simulink model "afe_abc_inv_psm_2mods"  (R2025b)
settings: Solver=ode1  StartTime=0.0  StopTime=simlength  FixedStep=tc  MaxStep=tc
values from neighbouring files (symbols this model uses):
  Adrso = eye(2) + Arso*ts_afe    [init_model.m]
  afe_pwm_phase_shift_mod1 = 0    [init_model.m]
  afe_pwm_phase_shift_mod2 = 0    [init_model.m]
  Aresd = eye(2) + Ares*ts_afe    [init_model.m]
  Bresd = Bres*ts_afe    [init_model.m]
  Cresd = Cres    [init_model.m]
  Crso = [1 0]    [init_model.m]
  CTRPIFF_CLIP_RELEASE = 0.001    [init_model.m]
  dead_time_AFE = 3e-6    (= 3e-06)    [init_model.m]
  dead_time_INV = 3e-6    (= 3e-06)    [init_model.m]
  deepNEGeta = 0.5    [init_model.m]
  deepNEGxi = 0    [init_model.m]
  deepPOSxi = 0.5    [init_model.m]
  emf_fb_p = 0.2    [init_model.m]
  emf_fb_p_ccaller_1 = emf_fb_p    (= 0.2)    [init_model.m]
  emf_fb_p_ccaller_2 = emf_fb_p    (= 0.2)    [init_model.m]
  emf_p = emf_fb_p*4/10    (= 0.08)    [init_model.m]
  emf_p_ccaller_1 = emf_fb_p_ccaller_1*4/10    (= 0.08)    [init_model.m]
  emf_p_ccaller_2 = emf_fb_p_ccaller_2*4/10    (= 0.08)    [init_model.m]
  fPWM_AFE = 4e3    (= 4000)    [init_model.m]
  fPWM_INV = fPWM_AFE    (= 4000)    [init_model.m]
  g0_161Hz = fcut_161Hz_flt * ts_afe * 2*pi    (= 0.126449104307)    [init_model.m]
  g0_1Hz = fcut_1Hz_flt * ts_afe * 2*pi    (= 0.000785398163397)    [init_model.m]
  g0_500Hz = fcut_500Hz_flt * ts_afe * 2*pi    (= 0.392699081699)    [init_model.m]
  g1_161Hz = 1 - g0_161Hz    (= 0.873550895693)    [init_model.m]
  g1_1Hz = 1 - g0_1Hz    (= 0.999214601837)    [init_model.m]
  g1_500Hz = 1 - g0_500Hz    (= 0.607300918301)    [init_model.m]
  i_grid_neg_eta_lim = 0.5    [init_model.m]
  i_grid_neg_eta_red_lim = 0.1    [init_model.m]
  i_grid_neg_xi_lim = 0.5    [init_model.m]
  i_grid_neg_xi_red_lim = 0.1    [init_model.m]
  i_grid_pos_eta_lim = 1    [init_model.m]
  i_grid_pos_eta_red_lim = 0.1    [init_model.m]
  id_lim = 0.35    [init_model.m]
  ieta_neg_ref_lim = 0.5    [init_model.m]
  ieta_pos_ref_lim = 1.0    (= 1)    [init_model.m]
  Igrid_phase_normalization_factor = 250e3/Vphase2/3/0.9*sqrt(2)    [init_model.m]
  inv_pwm_phase_shift_mod1 = 0    [init_model.m]
  iq_lim = 1.4    [init_model.m]
  ixi_pos_ref_lim = 1.6    [init_model.m]
  k_frt_ref = 2    [init_model.m]
  kg = Kobs(1)    [init_model.m]
  ki_afe = 45    [init_model.m]
  ki_align = 0.1    [init_model.m]
  ki_i = 18    [init_model.m]
  ki_rc_neg_grid = ki_rc_grid    (= 35)    [init_model.m]
  ki_rc_pos_grid = ki_rc_grid    (= 35)    [init_model.m]
  ki_vs = 35    [init_model.m]
  ki_w = 18    [init_model.m]
  kp_afe = 0.6    [init_model.m]
  kp_align = 0.6    [init_model.m]
  kp_i = 0.25    [init_model.m]
  kp_rc_neg_grid = kp_rc_grid    (= 0.35)    [init_model.m]
  kp_rc_pos_grid = kp_rc_grid    (= 0.35)    [init_model.m]
  kp_vs = 0.85    [init_model.m]
  kp_w = 2.5    [init_model.m]
  kw = Kobs(2)    [init_model.m]
  l1 = Kd(2)    [init_model.m]
  l2 = Kd(1)    [init_model.m]
  Ldrso = acker(Adrso',Crso',polesdrso)'    [init_model.m]
  lim_down_align = -0.2    [init_model.m]
  lim_up_align = 0.2    [init_model.m]
  mavarage_filter_frequency_base_order = 2    [init_model.m]
  motorc_m_scale = 2/3*Vdc_bez/ubez    [init_model.m]
  n1 = rms_perios/f_grid/ts_afe    [init_model.m]
  n10 = rms_perios/f_grid/ts_afe    [init_model.m]
  number_of_modules = 2    [init_model.m]
  omega_m_sim = omega_m_bez    [init_model.m]
  pll_i1 = 80    [init_model.m]
  pll_i1_ddsrt = pll_i1/2    (= 40)    [init_model.m]
  pll_p = 1    [init_model.m]
  pll_p_ddsrt = pll_p/2    (= 0.5)    [init_model.m]
  pll_p_frt = 0.2    [init_model.m]
  settle_time = 0.15    [init_model.m]
  simlength = 2    [init_model.m]
  start_time_LVRT = 2.0    (= 2)    [init_model.m]
  tc = ts_afe/200    (= 6.25e-07)    [init_model.m]
  time_aux_power_supply_fault = 1e3    (= 1000)    [init_model.m]
  time_gain_afe_module_1 = 1.0    (= 1)    [init_model.m]
  time_gain_afe_module_2 = 1.0    (= 1)    [init_model.m]
  time_gain_inv_module_1 = 1.0    (= 1)    [init_model.m]
  time_gain_inv_module_2 = 1.0    (= 1)    [init_model.m]
  time_phase_fault = 1e3    (= 1000)    [init_model.m]
  time_start_motor_control = 0.035    [init_model.m]
  transmission_delay = 125e-6*2    (= 0.00025)    [init_model.m]
  ts_afe = 1/fPWM_AFE/2    (= 0.000125)    [init_model.m]
  ts_inv = 1/fPWM_INV/2    (= 0.000125)    [init_model.m]
  Vdc_norm_ref = Vdc_ref/Vdc_nom    [init_model.m]
  Vdc_ref = 1070    [init_model.m]
  Vgrid_phase_normalization_factor = Vphase2*sqrt(2)    [init_model.m]
  w_grid = 2*pi*f_grid    [init_model.m]
undefined symbols (not defined in the file or in its folder): Amplitude_U, Amplitude_V, Amplitude_W, end_time_LVRT, ibez, La, Lb, Ld_norm, Lq_norm, Ls_norm, magnitude, omega_bez, omega_grid_emulator_nom, omega_grid_nom, omega_m_bez, Phase_shift, psi_bez, psi_m, psi_m_norm, rpm_base, rpm_bez, Rs, Rs_norm, t_ramp, tau_bez, torque_base, ubez, ugrid_factor, V_phase_normalization_factor, Vdc_bez, Vemu_ref_norm, vn_eta_pu, vn_xi_pu, vp_xi_pu
libraries: fl_lib x215, nesl_utility x107, simulink x22, cstblocks x20, threephase_inductor_lib x4, single_phase_transformer_lib x3, flexshaft_lib x1, psm x1
(part 12 of 19)

== system afe_abc_inv_psm_2mods/afe_abc_inv_psm_mod2/AFE_control/afe_control/grid_voltage_phase_lock_loops/DDSRF-PLL/pll_stageB ==
  u_grid_pos_xi : Inport
  u_grid_pos_eta : Inport  Port=2
  -2<x<2 : Saturate  UpperLimit=2  LowerLimit=-2
  Constant2 : Constant
  Constant3 : Constant  Value=0
  Constant4 : Constant  Value=omega_grid_nom
  Constant5 : Constant
  Constant6 : Constant  Value=-1
  Math Function : Math  Operator=magnitude^2  SignedPower=on
  Math Function2 : Math  Operator=magnitude^2  SignedPower=on
  Product{,1..3} (4 alike) : Product  RndMeth=Zero
  Sqrt : Sqrt
  Sum : Sum  Inputs=|-+
  Sum1 : Sum  Inputs=|-+
  Sum2 : Sum  Inputs=|++
  Sum3 : Sum  SaturateOnIntegerOverflow=on
  Sum4 : Sum  SaturateOnIntegerOverflow=on
  Sum5 : Sum  Inputs=++|
  Switch : Switch  Criteria=u2 > Threshold  SaturateOnIntegerOverflow=off  InputSameDT=off
  To Workspace5 : ToWorkspace  VariableName=vgrid_xi_pll_pos  SampleTime=-1
      settings: MaxDataPoints=Ns_afe
  To Workspace6 : ToWorkspace  VariableName=vgrid_eta_pll_pos  SampleTime=-1
      settings: MaxDataPoints=Ns_afe
  Unit Delay1 : UnitDelay  SampleTime=-1  HasFrameUpgradeWarning=on
  Unit Delay2 : UnitDelay  SampleTime=-1  HasFrameUpgradeWarning=on
  Unit Delay4 : UnitDelay  SampleTime=-1  HasFrameUpgradeWarning=on
  bounder1 : MATLAB Function  TreatAsAtomicUnit=on
  double_integrator_observer : Subsystem
  kp : Gain  Gain=pll_i1_ddsrt*ts_afe  SaturateOnIntegerOverflow=on  OutDataTypeStr=Inherit: Same as input  ParamDataTypeStr=Inherit: Same as input
  kp1 : Gain  Gain=pll_p_ddsrt  SaturateOnIntegerOverflow=on  OutDataTypeStr=Inherit: Same as input  ParamDataTypeStr=Inherit: Same as input
  kp2 : Gain  Gain=ts_afe  SaturateOnIntegerOverflow=on  OutDataTypeStr=Inherit: Same as input  ParamDataTypeStr=Inherit: Same as input
  gamma_grid_ddsrf_pll : Outport  VectorParamsAs1DForOutWhenUnconnected=off
  omega_grid_ddsrf_pll : Outport  Port=2  VectorParamsAs1DForOutWhenUnconnected=off
  wires:
  double_integrator_observer/1(omega_hat) -> omega_grid_ddsrf_pll/1
  Product/1 -> Sum/1
  Constant2/1 -> Sum/2
  Product1/1 -> Sum1/1
  Constant3/1 -> Sum1/2
  Math Function/1 -> Sum2/1
  Math Function2/1 -> Sum2/2
  Sum2/1 -> Sqrt/1
  Sum/1 -> Math Function/1
  Sum1/1 -> Switch/2, Math Function2/1
  Unit Delay4/1 -> Sum3/2
  Sum3/1 -> -2<x<2/1
  Sum4/1 -> bounder1/1(u)
  Unit Delay1/1 -> Sum4/2
  -2<x<2/1 -> Sum5/2, Unit Delay4/1  "i1"
  kp2/1 -> Sum4/1
  Constant4/1 -> Product2/2
  [Vgrid_unorm] -> Product/2, Product1/2
  Constant5/1 -> Switch/3
  Constant6/1 -> Switch/1
  Sqrt/1 -> Product3/1
  Switch/1 -> Product3/2
  kp/1 -> Sum3/1
  Sum5/1 -> Product2/1
  bounder1/1(y) -> Unit Delay2/1, Unit Delay1/1
  u_grid_pos_xi/1 -> Product/1, To Workspace5/1
  u_grid_pos_eta/1 -> To Workspace6/1, Product1/1
  Product2/1 -> kp2/1
  Product3/1 -> kp1/1, kp/1  "V l"
  kp1/1 -> Sum5/1
  Unit Delay2/1 -> double_integrator_observer/1(theta), gamma_grid_ddsrf_pll/1

== system afe_abc_inv_psm_2mods/afe_abc_inv_psm_mod2/AFE_control/afe_control/grid_voltage_phase_lock_loops/dq_pll/pll_stageA ==
  gamma_grid : Inport
  ug_abc : Inport  Port=2
  Demux : Demux  Outputs=3
  Math Function : Math  Operator=magnitude^2  SignedPower=on
  Math Function1 : Math  Operator=magnitude^2  SignedPower=on
  Reciprocal Sqrt : Sqrt  Operator=rSqrt
  Saturation : Saturate  UpperLimit=inf  LowerLimit=0.02
  Sum : Sum  Inputs=|++
  mormalization_and_transformation : Subsystem
  sequences : Subsystem
  u_grid_pos_xi : Outport  VectorParamsAs1DForOutWhenUnconnected=off
  u_grid_pos_eta : Outport  Port=2  VectorParamsAs1DForOutWhenUnconnected=off
  tag scope: Vgrid_unorm_mod2=global
  wires:
  Saturation/1 -> Reciprocal Sqrt/1
  Math Function/1 -> Sum/1
  Sum/1 -> Saturation/1
  Reciprocal Sqrt/1 -> [Vgrid_unorm_mod2]
  mormalization_and_transformation/2(ug_beta) -> sequences/2(u_grid_beta), Math Function1/1
  mormalization_and_transformation/1(ug_alpha) -> sequences/1(u_grid_alpha), Math Function/1
  Math Function1/1 -> Sum/2
  sequences/2(u_grid_pos_eta) -> u_grid_pos_eta/1
  sequences/1(u_grid_pos_xi) -> u_grid_pos_xi/1
  gamma_grid/1 -> sequences/3(gamma_grid)
  Demux/3 -> mormalization_and_transformation/3(ug_c)
  Demux/2 -> mormalization_and_transformation/2(ug_b)
  Demux/1 -> mormalization_and_transformation/1(ug_a)
  ug_abc/1 -> Demux/1

== system afe_abc_inv_psm_2mods/afe_abc_inv_psm_mod2/AFE_control/afe_control/grid_voltage_phase_lock_loops/dq_pll/pll_stageB ==
  u_grid_pos_xi : Inport
  u_grid_pos_eta : Inport  Port=2
  -2<x<2 : Saturate  UpperLimit=2  LowerLimit=-2
  Constant4 : Constant  Value=omega_grid_nom
  Product1 : Product  RndMeth=Zero
  Product2 : Product  RndMeth=Zero
  Sum3 : Sum  SaturateOnIntegerOverflow=on
  Sum4 : Sum  SaturateOnIntegerOverflow=on
  Sum5 : Sum  Inputs=++|
  Unit Delay1 : UnitDelay  SampleTime=-1  HasFrameUpgradeWarning=on
  Unit Delay2 : UnitDelay  SampleTime=-1  HasFrameUpgradeWarning=on
  Unit Delay4 : UnitDelay  SampleTime=-1  HasFrameUpgradeWarning=on
  bounder1 : MATLAB Function  TreatAsAtomicUnit=on
  double_integrator_observer : Subsystem
  kp : Gain  Gain=pll_i1*ts_afe  SaturateOnIntegerOverflow=on  OutDataTypeStr=Inherit: Same as input  ParamDataTypeStr=Inherit: Same as input
  kp1 : Gain  Gain=1/omega_grid_nom  SaturateOnIntegerOverflow=on  OutDataTypeStr=Inherit: Same as input  ParamDataTypeStr=Inherit: Same as input
  kp2 : Gain  Gain=ts_afe  SaturateOnIntegerOverflow=on  OutDataTypeStr=Inherit: Same as input  ParamDataTypeStr=Inherit: Same as input
  scheduled-p-gain : Subsystem
      settings: PortSchema="{\"entries\":[{\"content\":{\"sides\":[{\"content\":{},\"type\":\"ConnectorPlacement.EquallySpacedRectSide\",\"uuid\":\"88e64df2-a299-4c1b-9bac-7a615cd04a00\"},{\"content\":{\"side\":\"RIGHT\"},\"type\":\"ConnectorPlacement.EquallySpacedRectSide\",\"uuid\":\"ef1d7318-b0e2-4e96-bf99-c42bb4ec5202\"},{\"content\":{\"connectorIds\":[\"In1\"],\"side\":\"TOP\"},\"type\":\"ConnectorPlacement.EquallySpacedRectSide\",\"uuid\":\"96582c59-f6c8-40f1-b3cf-394cc239c4b2\"},{\"content\":{\"connectorIds\":[\"Out1\"],\"side\":\"BOTTOM\"},\"type\":\"ConnectorPlacement.EquallySpacedRectSide\",\"uuid\":\"9ac5cd0d-958f-4b67-b4ea-90856a0aa038\"}]},\"type\":\"ConnectorPlacement.EquallySpacedConnector\",\"uuid\":\"ca37db80-6b94-4315-bd9c-66307567cd1f\"}],\"packageUris\":[\"http://schema.mathworks.com/mf0/Connector/R2020b\"],\"version\":\"1.0\"}"
  gamma_grid_pll : Outport  VectorParamsAs1DForOutWhenUnconnected=off
  omega_grid_pll : Outport  Port=2  VectorParamsAs1DForOutWhenUnconnected=off
  wires:
  double_integrator_observer/1(omega_hat) -> kp1/1
  Unit Delay2/1 -> gamma_grid_pll/1, double_integrator_observer/1(theta)
  scheduled-p-gain/1(Out2) -> Sum5/1
  Product1/1 -> kp/1, scheduled-p-gain/1(In1)  "V l"
  Product2/1 -> kp2/1
  u_grid_pos_eta/1 -> Product1/1
  bounder1/1(y) -> Unit Delay2/1, Unit Delay1/1
  Sum5/1 -> Product2/1
  kp/1 -> Sum3/1
  [Vgrid_unorm_mod2] -> Product1/2
  Constant4/1 -> Product2/2
  kp2/1 -> Sum4/1
  -2<x<2/1 -> Unit Delay4/1, Sum5/2  "i1"
  Unit Delay1/1 -> Sum4/2
  Sum4/1 -> bounder1/1(u)
  Sum3/1 -> -2<x<2/1
  Unit Delay4/1 -> Sum3/2
  kp1/1 -> omega_grid_pll/1

== system afe_abc_inv_psm_2mods/afe_abc_inv_psm_mod2/AFE_control/afe_control/grid_voltage_phase_lock_loops/dq_pll_ccaller/first_harmonic_tracker_phase_u ==
  u : Inport
  Bus Selector : BusSelector  OutputSignals=output_pu_hat
  C Caller : CCaller  FunctionName=first_harmonic_tracker_process_simulink  PortSpecificationStruct="%)30     .    V @   8    (     @         %    \"     4    !     0         %  0 \"0    $    _    07)G3F%M90  4&]R=$YA;64 4V-O<&4     26YD97@     5'EP90      4VEZ90      27-';&]B86P   X    P    !@    @    $          4    (     0    ,    !         !   P!O=70 #@   #     &    \"     0         !0    @    !     P    $         $  # &]U=  .    .     8    (    !          %    \"     $    &     0         0   ...(+2669 chars)"
  Constant : Constant  Value=ts_afe
  Constant1 : Constant  Value=6
  Data Type Conversion1 : DataTypeConversion  OutDataTypeStr=single  SaturateOnIntegerOverflow=off  RndMeth=Floor
  Data Type Conversion2 : DataTypeConversion  OutDataTypeStr=single  SaturateOnIntegerOverflow=off  RndMeth=Floor
  Data Type Conversion3 : DataTypeConversion  OutDataTypeStr=uint8  SaturateOnIntegerOverflow=off  RndMeth=Floor
  Data Type Conversion4 : DataTypeConversion  OutDataTypeStr=double  SaturateOnIntegerOverflow=off  RndMeth=Floor
  Data Type Conversion5 : DataTypeConversion  OutDataTypeStr=uint8  SaturateOnIntegerOverflow=off  RndMeth=Floor
  Step : Step  Time=0.0125  Before=1  After=0
  u_hat : Outport
  wires:
  Constant1/1 -> Data Type Conversion5/1
  Data Type Conversion5/1 -> C Caller/4
  Constant/1 -> Data Type Conversion1/1
  u/1 -> Data Type Conversion2/1
  Step/1 -> Data Type Conversion3/1
  Bus Selector/1 -> Data Type Conversion4/1  "<output_pu_hat>"
  C Caller/1 -> Bus Selector/1
  Data Type Conversion2/1 -> C Caller/2
  Data Type Conversion1/1 -> C Caller/3
  Data Type Conversion3/1 -> C Caller/1
  Data Type Conversion4/1 -> u_hat/1

== system afe_abc_inv_psm_2mods/afe_abc_inv_psm_mod2/AFE_control/afe_control/grid_voltage_phase_lock_loops/dq_pll_ccaller/first_harmonic_tracker_phase_v ==
  u : Inport
  Bus Selector : BusSelector  OutputSignals=output_pu_hat
  C Caller : CCaller  FunctionName=first_harmonic_tracker_process_simulink  PortSpecificationStruct="%)30     .    V @   8    (     @         %    \"     4    !     0         %  0 \"0    $    _    07)G3F%M90  4&]R=$YA;64 4V-O<&4     26YD97@     5'EP90      4VEZ90      27-';&]B86P   X    P    !@    @    $          4    (     0    ,    !         !   P!O=70 #@   #     &    \"     0         !0    @    !     P    $         $  # &]U=  .    .     8    (    !          %    \"     $    &     0         0   ...(+2669 chars)"
  Constant : Constant  Value=ts_afe
  Constant1 : Constant  Value=8
  Data Type Conversion1 : DataTypeConversion  OutDataTypeStr=single  SaturateOnIntegerOverflow=off  RndMeth=Floor
  Data Type Conversion2 : DataTypeConversion  OutDataTypeStr=single  SaturateOnIntegerOverflow=off  RndMeth=Floor
  Data Type Conversion3 : DataTypeConversion  OutDataTypeStr=uint8  SaturateOnIntegerOverflow=off  RndMeth=Floor
  Data Type Conversion4 : DataTypeConversion  OutDataTypeStr=double  SaturateOnIntegerOverflow=off  RndMeth=Floor
  Data Type Conversion5 : DataTypeConversion  OutDataTypeStr=uint8  SaturateOnIntegerOverflow=off  RndMeth=Floor
  Step : Step  Time=0.0125  Before=1  After=0
  u_hat : Outport
  wires:
  Data Type Conversion4/1 -> u_hat/1
  Data Type Conversion3/1 -> C Caller/1
  Data Type Conversion1/1 -> C Caller/3
  Data Type Conversion2/1 -> C Caller/2
  C Caller/1 -> Bus Selector/1
  Bus Selector/1 -> Data Type Conversion4/1  "<output_pu_hat>"
  Step/1 -> Data Type Conversion3/1
  u/1 -> Data Type Conversion2/1
  Constant/1 -> Data Type Conversion1/1
  Data Type Conversion5/1 -> C Caller/4
  Constant1/1 -> Data Type Conversion5/1

== system afe_abc_inv_psm_2mods/afe_abc_inv_psm_mod2/AFE_control/afe_control/grid_voltage_phase_lock_loops/dq_pll_ccaller/first_harmonic_tracker_phase_w ==
  u : Inport
  Bus Selector : BusSelector  OutputSignals=output_pu_hat
  C Caller : CCaller  FunctionName=first_harmonic_tracker_process_simulink  PortSpecificationStruct="%)30     .    V @   8    (     @         %    \"     4    !     0         %  0 \"0    $    _    07)G3F%M90  4&]R=$YA;64 4V-O<&4     26YD97@     5'EP90      4VEZ90      27-';&]B86P   X    P    !@    @    $          4    (     0    ,    !         !   P!O=70 #@   #     &    \"     0         !0    @    !     P    $         $  # &]U=  .    .     8    (    !          %    \"     $    &     0         0   ...(+2669 chars)"
  Constant : Constant  Value=ts_afe
  Constant1 : Constant  Value=10
  Data Type Conversion1 : DataTypeConversion  OutDataTypeStr=single  SaturateOnIntegerOverflow=off  RndMeth=Floor
  Data Type Conversion2 : DataTypeConversion  OutDataTypeStr=single  SaturateOnIntegerOverflow=off  RndMeth=Floor
  Data Type Conversion3 : DataTypeConversion  OutDataTypeStr=uint8  SaturateOnIntegerOverflow=off  RndMeth=Floor
  Data Type Conversion4 : DataTypeConversion  OutDataTypeStr=double  SaturateOnIntegerOverflow=off  RndMeth=Floor
  Data Type Conversion5 : DataTypeConversion  OutDataTypeStr=uint8  SaturateOnIntegerOverflow=off  RndMeth=Floor
  Step : Step  Time=0.0125  Before=1  After=0
  u_hat : Outport
  wires:
  Constant1/1 -> Data Type Conversion5/1
  Data Type Conversion5/1 -> C Caller/4
  Constant/1 -> Data Type Conversion1/1
  u/1 -> Data Type Conversion2/1
  Step/1 -> Data Type Conversion3/1
  Bus Selector/1 -> Data Type Conversion4/1  "<output_pu_hat>"
  C Caller/1 -> Bus Selector/1
  Data Type Conversion2/1 -> C Caller/2
  Data Type Conversion1/1 -> C Caller/3
  Data Type Conversion3/1 -> C Caller/1
  Data Type Conversion4/1 -> u_hat/1

== system afe_abc_inv_psm_2mods/afe_abc_inv_psm_mod2/AFE_control/afe_control/grid_voltage_sequences/voltage_sequence_avg/average_filter_ccaller ==
  v_grid_pos_xi : Inport
  v_grid_pos_eta : Inport  Port=2
  v_grid_neg_xi : Inport  Port=3
  v_grid_neg_eta : Inport  Port=4
  Gain : Gain  Gain=w_grid
  Moving Average Filter1 : Subsystem
  Moving Average Filter2 : Subsystem
  Moving Average Filter3 : Subsystem
  Moving Average Filter4 : Subsystem
  v_grid_pos_xi_avg : Outport
  v_grid_pos_eta_avg : Outport  Port=2
  v_grid_neg_xi_avg : Outport  Port=3
  v_grid_neg_eta_avg : Outport  Port=4
  wires:
  v_grid_pos_eta/1 -> Moving Average Filter2/1(In2)
  Moving Average Filter1/1(xi) -> v_grid_pos_xi_avg/1
  Moving Average Filter4/1(xi) -> v_grid_neg_eta_avg/1
  Moving Average Filter3/1(xi) -> v_grid_neg_xi_avg/1
  v_grid_neg_eta/1 -> Moving Average Filter4/1(In2)
  v_grid_neg_xi/1 -> Moving Average Filter3/1(In2)
  v_grid_pos_xi/1 -> Moving Average Filter1/1(In2)
  [omega_grid_pll_mod2] -> Gain/1
  Moving Average Filter2/1(xi) -> v_grid_pos_eta_avg/1
  Gain/1 -> Moving Average Filter3/2(In3), Moving Average Filter4/2(In3), Moving Average Filter2/2(In3), Moving Average Filter1/2(In3)

== system afe_abc_inv_psm_2mods/afe_abc_inv_psm_mod2/AFE_control/afe_control/grid_voltage_sequences/voltage_sequence_avg/average_filter_simulink ==
  v_grid_pos_xi : Inport
  v_grid_pos_eta : Inport  Port=2
  v_grid_neg_xi : Inport  Port=3
  v_grid_neg_eta : Inport  Port=4
  moving_avarage_1 : Subsystem
  moving_avarage_2 : Subsystem
  moving_avarage_3 : Subsystem
  moving_avarage_4 : Subsystem
  v_grid_pos_xi_avg : Outport
  v_grid_pos_eta_avg : Outport  Port=2
  v_grid_neg_xi_avg : Outport  Port=3
  v_grid_neg_eta_avg : Outport  Port=4
  wires:
  moving_avarage_4/1(y) -> v_grid_neg_eta_avg/1  "v_grid_neg_eta_avg"
  moving_avarage_3/1(y) -> v_grid_neg_xi_avg/1  "v_grid_neg_xi_avg"
  moving_avarage_2/1(y) -> v_grid_pos_eta_avg/1  "v_grid_pos_eta_avg"
  moving_avarage_1/1(y) -> v_grid_pos_xi_avg/1  "v_grid_pos_xi_avg"
  v_grid_pos_eta/1 -> moving_avarage_2/1(u)
  v_grid_neg_eta/1 -> moving_avarage_4/1(u)
  v_grid_pos_xi/1 -> moving_avarage_1/1(u)
  v_grid_neg_xi/1 -> moving_avarage_3/1(u)

== system afe_abc_inv_psm_2mods/afe_abc_inv_psm_mod2/AFE_control/afe_control/phase_compensation_1/alignment_ctrl/pi ==
  u_ref : Inport
  u : Inport  Port=2
  1/Ti : Gain  Gain=kp  SaturateOnIntegerOverflow=on  OutDataTypeStr=Inherit: Same as input  ParamDataTypeStr=Inherit: Same as input
  Saturation : Saturate  UpperLimit=lim_up  LowerLimit=lim_down
  Sum1 : Sum  Inputs=+++  SaturateOnIntegerOverflow=on
  Sum2 : Sum  Inputs=-+  SaturateOnIntegerOverflow=on
  Sum3 : Sum  Inputs=-+  SaturateOnIntegerOverflow=on
  Unit Delay4 : UnitDelay  SampleTime=-1  HasFrameUpgradeWarning=on
  kp : Gain  Gain=ki  SaturateOnIntegerOverflow=on  OutDataTypeStr=Inherit: Same as input  ParamDataTypeStr=Inherit: Same as input
  y : Outport
  wires:
  1/Ti/1 -> Sum1/1, Sum3/1
  kp/1 -> Sum1/2
  Sum3/1 -> Unit Delay4/1
  Unit Delay4/1 -> Sum1/3
  u_ref/1 -> Sum2/2
  u/1 -> Sum2/1
  Sum2/1 -> kp/1, 1/Ti/1
  Sum1/1 -> Saturation/1
  Saturation/1 -> Sum3/2, y/1

== system afe_abc_inv_psm_2mods/afe_abc_inv_psm_mod2/INV_control/inverter_control/current_ctrl/bemf_observer/bemf_observer ==
  ialpha_pu : Inport
  ibeta_pu : Inport  Port=2
  ualpha_pu : Inport  Port=3
  ubeta_pu : Inport  Port=4
  udc_pu : Inport  Port=5
  Gain : Gain  Gain=psi_m_norm
  Gain1 : Gain  Gain=psi_m_norm
  Trigonometric Function : Trigonometry  Operator=cos
  Trigonometric Function1 : Trigonometry
  double_integrator_observer : Subsystem
  psi_alpha_hat : Subsystem
  psi_beta_hat : Subsystem
  theta_bemf_hat : Subsystem
  omega_pu : Outport
  theta_hat : Outport  Port=2
  tag scope: psi_r_alpha_hat_mod2=global, psi_r_alpha_pu_hat_mod2=global, psi_r_beta_hat_mod2=global, psi_r_beta_pu_hat_mod2=global, psi_r_m_alpha_mod2=global, psi_r_m_beta_mod2=global, theta_bemf_hat_mod2=global
  wires:
  udc_pu/1 -> psi_alpha_hat/3(udc), psi_beta_hat/3(udc)
  [psi_r_beta_hat_mod2] -> [psi_r_beta_pu_hat_mod2]
  [psi_r_alpha_hat_mod2] -> [psi_r_alpha_pu_hat_mod2]
  double_integrator_observer/2(theta_hat) -> theta_hat/1
  double_integrator_observer/1(omega_pu_hat) -> omega_pu/1
  [theta_bemf_hat_mod2] -> double_integrator_observer/1(theta)
  theta_bemf_hat/1(theta_emf_hat) -> [theta_bemf_hat_mod2]
  Gain1/1 -> [psi_r_m_beta_mod2]
  Gain/1 -> [psi_r_m_alpha_mod2]
  [theta_hat_mod2] -> Trigonometric Function1/1, Trigonometric Function/1
  ubeta_pu/1 -> psi_beta_hat/1(ubeta)
  ualpha_pu/1 -> psi_alpha_hat/1(ualpha)
  [psi_r_beta_hat_mod2] -> theta_bemf_hat/2(psi_r_beta_hat)
  [psi_r_alpha_hat_mod2] -> theta_bemf_hat/1(psi_r_alpha_hat)
  psi_beta_hat/2(psi_r_beta_hat) -> [psi_r_beta_hat_mod2]
  psi_alpha_hat/2(psi_r_alpha_hat) -> [psi_r_alpha_hat_mod2]
  ibeta_pu/1 -> psi_beta_hat/2(ibeta)
  ialpha_pu/1 -> psi_alpha_hat/2(ialpha)
  Trigonometric Function1/1 -> Gain1/1
  Trigonometric Function/1 -> Gain/1

== system afe_abc_inv_psm_2mods/afe_abc_inv_psm_mod2/INV_control/inverter_control/current_ctrl/bemf_observer/bemf_observer_ccaller ==
  ialpha_pu : Inport
  ibeta_pu : Inport  Port=2
  ualpha_pu : Inport  Port=3
  ubeta_pu : Inport  Port=4
  udc_pu : Inport  Port=5
  Bus Selector : BusSelector  OutputSignals=omega_pu_hat,theta_hat
  C Caller : CCaller  FunctionName=bemf_obsv_process_simulink  PortSpecificationStruct="%)30     .    N\"8   8    (     @         %    \"    !8    !     0         %  0 \"0    $    _    07)G3F%M90  4&]R=$YA;64 4V-O<&4     26YD97@     5'EP90      4VEZ90      27-';&]B86P   X    P    !@    @    $          4    (     0    ,    !         !   P!O=70 #@   #     &    \"     0         !0    @    !     P    $         $  # &]U=  .    .     8    (    !          %    \"     $    &     0         0  ...(+12985 chars)"
  Constant : Constant  Value=ts_inv
  Constant1 : Constant  Value=emf_fb_p_ccaller_1
  Constant10 : Constant  Value=emf_fb_p_ccaller_2
  Constant11 : Constant  Value=emf_p_ccaller_2
  Constant12 : Constant  Value=0
  Constant13 : Constant  Value=0
  Constant14 : Constant
  Constant2 : Constant  Value=emf_p_ccaller_1
  Constant3 : Constant  Value=omega_bez
  Constant4 : Constant  Value=motorc_m_scale
  Constant5 : Constant  Value=Rs_norm
  Constant6 : Constant  Value=Ls_norm
  Constant7 : Constant  Value=psi_m_norm
  Constant8 : Constant  Value=kw
  Constant9 : Constant  Value=kg
  Data Type Conversion{,1..2,4..6,9..22} (20 alike) : DataTypeConversion  OutDataTypeStr=single  SaturateOnIntegerOverflow=off  RndMeth=Floor
  Data Type Conversion3 : DataTypeConversion  OutDataTypeStr=double  SaturateOnIntegerOverflow=off  RndMeth=Floor
  Data Type Conversion7 : DataTypeConversion  OutDataTypeStr=double  SaturateOnIntegerOverflow=off  RndMeth=Floor
  Data Type Conversion8 : DataTypeConversion  OutDataTypeStr=uint8  SaturateOnIntegerOverflow=off  RndMeth=Floor
  Reset Trigger : Subsystem
  omega_pu : Outport
  theta_hat : Outport  Port=2
  wires:
  udc_pu/1 -> Data Type Conversion5/1
  Reset Trigger/1(Out1) -> Data Type Conversion8/1
  ualpha_pu/1 -> Data Type Conversion/1
  ubeta_pu/1 -> Data Type Conversion1/1
  ialpha_pu/1 -> Data Type Conversion2/1
  ibeta_pu/1 -> Data Type Conversion4/1
  Constant/1 -> Data Type Conversion6/1
  Constant1/1 -> Data Type Conversion9/1
  Constant2/1 -> Data Type Conversion10/1
  Constant10/1 -> Data Type Conversion19/1
  Constant11/1 -> Data Type Conversion18/1
  Constant3/1 -> Data Type Conversion11/1
  Constant4/1 -> Data Type Conversion12/1
  Constant5/1 -> Data Type Conversion13/1
  Constant6/1 -> Data Type Conversion14/1
  Constant7/1 -> Data Type Conversion15/1
  Constant8/1 -> Data Type Conversion16/1
  Constant9/1 -> Data Type Conversion17/1
  Constant12/1 -> Data Type Conversion20/1
  Constant13/1 -> Data Type Conversion21/1
  Constant14/1 -> Data Type Conversion22/1
  Data Type Conversion22/1 -> C Caller/21
  Data Type Conversion21/1 -> C Caller/20
  Data Type Conversion20/1 -> C Caller/19
  Data Type Conversion17/1 -> C Caller/18
  Data Type Conversion16/1 -> C Caller/17
  Data Type Conversion15/1 -> C Caller/16
  Data Type Conversion14/1 -> C Caller/15
  Data Type Conversion13/1 -> C Caller/14
  Data Type Conversion12/1 -> C Caller/13
  Data Type Conversion11/1 -> C Caller/12
  Data Type Conversion18/1 -> C Caller/11
  Data Type Conversion19/1 -> C Caller/10
  Data Type Conversion10/1 -> C Caller/9
  Data Type Conversion9/1 -> C Caller/8
  Data Type Conversion8/1 -> C Caller/1
  Data Type Conversion3/1 -> theta_hat/1  "theta_hat"
  Data Type Conversion7/1 -> omega_pu/1  "omega_pu"
  Bus Selector/1 -> Data Type Conversion7/1  "<omega_pu_hat>"
  Bus Selector/2 -> Data Type Conversion3/1  "<theta_hat>"
  Data Type Conversion6/1 -> C Caller/7
  Data Type Conversion2/1 -> C Caller/4
  Data Type Conversion4/1 -> C Caller/5
  Data Type Conversion1/1 -> C Caller/3
  C Caller/1 -> Bus Selector/1  "out"
  Data Type Conversion/1 -> C Caller/2
  Data Type Conversion5/1 -> C Caller/6

== system afe_abc_inv_psm_2mods/afe_abc_inv_psm_mod2/INV_control/inverter_control/current_ctrl/bemf_observer/phase_fault ==
  double_integrator_observer : Subsystem
  phase_fault : Subsystem
  omega_pu_encoder : Outport
  theta_hat_encoder : Outport  Port=2
  wires:
  double_integrator_observer/1(omega_pu_hat) -> omega_pu_encoder/1  "omega_pu_encoder"
  phase_fault/1(theta) -> double_integrator_observer/1(theta)
  double_integrator_observer/2(theta_hat) -> theta_hat_encoder/1  "theta_hat_encoder"
  [theta_elec_psm] -> phase_fault/1(theta_pmsm)  "theta_pmsm"

== system afe_abc_inv_psm_2mods/afe_abc_inv_psm_mod2/INV_control/inverter_control/current_ctrl/current_ctrl/MTPA _mod1 ==
  iq_ref : Inport
  Gain1 : Gain  Gain=1/(Ld_norm - Lq_norm)/2
  Gain2 : Gain  Gain=1/(Ld_norm - Lq_norm)/2
  Gain3 : Gain  Gain=-1
  Math Function1 : Math  Operator=magnitude^2  SignedPower=on
  Math Function4 : Math  Operator=magnitude^2  SignedPower=on
  Sqrt : Sqrt
  Sum : Sum  Inputs=|++
  Sum1 : Sum  Inputs=|-+
  id_ref_pu < x < 0 : Saturate  UpperLimit=0  LowerLimit=-id_lim
  Id_ref_mtpa : Outport  VectorParamsAs1DForOutWhenUnconnected=off
  wires:
  Gain3/1 -> id_ref_pu < x < 0/1
  [omega_hat_pu_mod2] -> Gain2/1, Gain1/1
  Gain2/1 -> Sum1/1
  iq_ref/1 -> Math Function1/1
  Sqrt/1 -> Sum1/2
  Sum/1 -> Sqrt/1
  Gain1/1 -> Math Function4/1
  Math Function1/1 -> Sum/2
  Math Function4/1 -> Sum/1
  id_ref_pu < x < 0/1 -> Id_ref_mtpa/1
  Sum1/1 -> Gain3/1
